simulink model "Position"  (R2020a)
settings: Solver=ode15s  StartTime=0.0  StopTime=0.2  RelTol=1e-3
values from neighbouring files (symbols this model uses):
  b = 3.5077e-06    [pos.mat]
  J = 3.2284e-06    [pos.mat]
  Ke = 0.0274    [pos.mat]
  Kt = 0.0274    [pos.mat]
  L = 2.75e-06    [pos.mat]
  R = 4    [pos.mat]
settings Model: Creator=Admin  LastModifiedBy=Admin

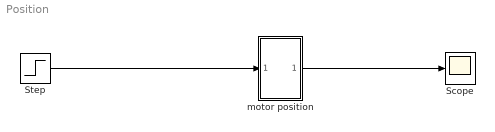
== system Position ==
  Scope : Scope
  Step : Step  Time=0  SampleTime=0
  motor position : Subsystem
  wires:
  Step/1 -> motor position/1(In1)
  motor position/1(Out1) -> Scope/1

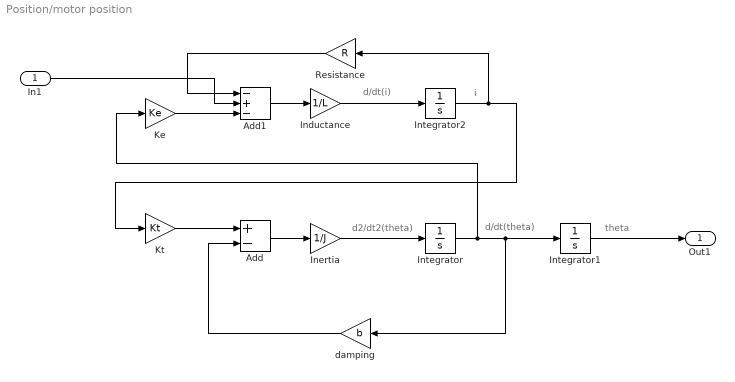
== system Position/motor position ==
  note: d/dt(i)
  note: i
  note: d/dt(theta)
  note: theta
  note: d2/dt2(theta)
  In1 : Inport
  Add : Sum  Inputs=+-
  Add1 : Sum  Inputs=-+-
  Inductance : Gain  Gain=1/L
  Inertia : Gain  Gain=1/J
  Integrator : Integrator
  Integrator1 : Integrator
  Integrator2 : Integrator
  Ke : Gain  Gain=Ke
  Kt : Gain  Gain=Kt
  Resistance : Gain  Gain=R
  damping : Gain  Gain=b
  Out1 : Outport
  wires:
  Ke/1 -> Add1/3
  Integrator2/1 -> Resistance/1, Kt/1
  Add1/1 -> Inductance/1
  Inductance/1 -> Integrator2/1
  Resistance/1 -> Add1/1
  damping/1 -> Add/2
  Kt/1 -> Add/1
  Inertia/1 -> Integrator/1
  Integrator/1 -> Ke/1, damping/1, Integrator1/1
  Add/1 -> Inertia/1
  Integrator1/1 -> Out1/1
  In1/1 -> Add1/2
